simulink model "closedloop"  (Simulink 8.5)
settings: Solver=ode3  StartTime=0.0  StopTime=60  FixedStep=1e-2  RelTol=1e-3
undefined symbols (not defined in the file): C, I, wn, xi
libraries: simulink x1
settings Model: Creator=henrik_2  LastModifiedBy=hg35a  CovSFcnEnable=off
settings DataIOCC: SignalLoggingName=sigsOut
settings OptimizationCC: InitFltsAndDblsToZero=on
settings DebuggingCC: SaveWithParameterizedLinksMsg=none  SignalResolutionControl=TryResolveAllWithWarning  MultiTaskDSMMsg=warning  MultiTaskCondExecSysMsg=none  FcnCallInpInsideContextMsg=UseLocalSettings
settings HardwareCC: TargetUnknown=on
settings GRTTargetCC: TargetFcnLib=ansi_tfl_tmw.mat  ModelReferenceCompliant=off  MatFileLogging=off

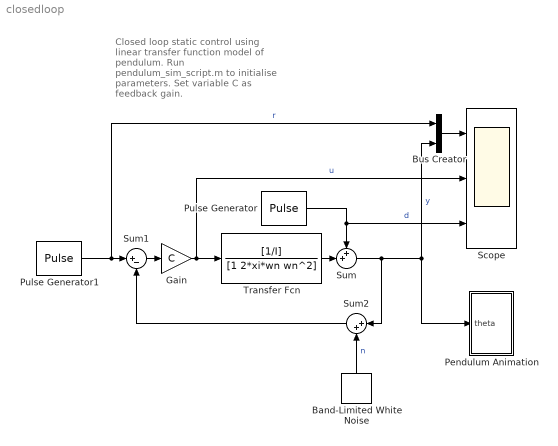
== system closedloop ==
  note: Closed loop static control
      | using linear transfer function
      | model of pendulum.
      | Run pendulum_sim_script.m to
      | initialise parameters.
      | Set variable C as feedback gain.
  Band-Limited White Noise : simulink/Sources/Band-Limited White Noise  Cov=[0.000001]*0  Ts=0.01  seed=[23341]
  Bus Creator : BusCreator  Inputs=2
  Gain : Gain  Gain=C  SaturateOnIntegerOverflow=on  OutDataTypeStr=Inherit: Same as input  ParamDataTypeStr=Inherit: Same as input
  Pendulum Animation : Subsystem
  Pulse Generator : DiscretePulseGenerator  PulseType=Time based  Amplitude=0.1*0  Period=30  PulseWidth=50  PhaseDelay=15
  Pulse Generator1 : DiscretePulseGenerator  PulseType=Time based  Amplitude=0.3  Period=10  PulseWidth=50
  Scope : Scope  NumInputPorts=3
      settings: ShowLegends=on  YMin=-0.4~-400~0  YMax=0.6~400~0.1
  Sum : Sum  Inputs=++|  SaturateOnIntegerOverflow=on
  Sum1 : Sum  Inputs=|+-  SaturateOnIntegerOverflow=on
  Sum2 : Sum  Inputs=|++  SaturateOnIntegerOverflow=on
  Transfer Fcn : TransferFcn  Numerator=[1/I]  Denominator=[1 2*xi*wn wn^2]
  wires:
  Gain/1 -> Scope/2, Transfer Fcn/1  "u"
  Transfer Fcn/1 -> Sum/2
  Pulse Generator/1 -> Sum/1, Scope/3  "d"
  Pulse Generator1/1 -> Bus Creator/1, Sum1/1  "r"
  Bus Creator/1 -> Scope/1
  Sum/1 -> Bus Creator/2, Pendulum Animation/1(theta), Sum2/1  "y"
  Sum1/1 -> Gain/1
  Sum2/1 -> Sum1/2
  Band-Limited White Noise/1 -> Sum2/2  "n"

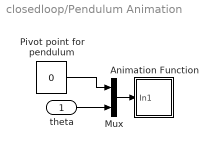
== system closedloop/Pendulum Animation ==
  theta : Inport
  Animation Function : Subsystem  mask(Animation Block){ts=0.01}
      mask prompts: ts "Sample time:"
      mask Display: plot([.1,.9],[.9,.9],[.5,.2],[.9,.25],[.475,.475,.525,.525,.475],[.875,.925,.925,.875,.875])
  Mux : Mux  Inputs=2
  Pivot point for pendulum : Constant  Value=0
  wires:
  Mux/1 -> Animation Function/1(In1)
  Pivot point for pendulum/1 -> Mux/1
  theta/1 -> Mux/2

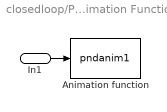
== system closedloop/Pendulum Animation/Animation Function ==
  In1 : Inport
  Animation function : S-Function  FunctionName=pndanim1  Parameters=ts
      settings: DeleteFcn=if ~isempty(findobj('type','figure','name','simppend Animation'));close('simppend Animation'); end;
  wires:
  In1/1 -> Animation function/1
